simulink model "LQR_1"  (R2022a)
settings: Solver=VariableStepAuto  StartTime=0.0  StopTime=60  RelTol=1e-3
values from neighbouring files (symbols this model uses):
  A = double(A)    [LQR.m]
  B = double(B)    [LQR.m]
undefined symbols (not defined in the file or in its folder): K
libraries: cstblocks x2, simulink x1
settings Model: Creator=Shiva  LastModifiedBy=Shiva

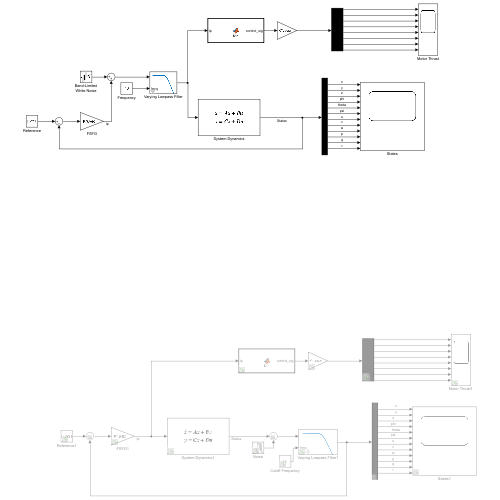
[thumbnail: Simulink's stored preview of the top-level diagram]
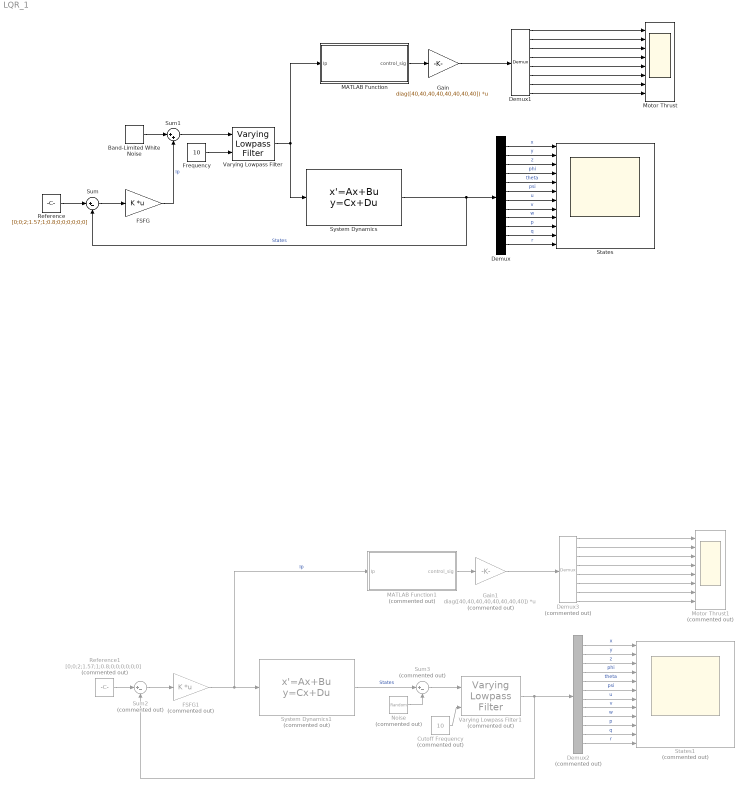
== system LQR_1 ==
  Band-Limited White Noise : simulink/Sources/Band-Limited White Noise  Cov=[0.1]  Ts=0.1  seed=[23341]
  Cutoff Frequency : Constant  Commented=on  Value=10
  Demux : Demux  Outputs=12
  Demux1 : Demux  Outputs=8
  Demux2 : Demux  Commented=on  Outputs=12
  Demux3 : Demux  Commented=on  Outputs=8
  FSFG : Gain  Gain=K  Multiplication=Matrix(K*u) (u vector)
  FSFG1 : Gain  Commented=on  Gain=K  Multiplication=Matrix(K*u) (u vector)
  Frequency : Constant  Value=10
  Gain : Gain  Gain=diag([40,40,40,40,40,40,40,40])  Multiplication=Matrix(K*u) (u vector)
  Gain1 : Gain  Commented=on  Gain=diag([40,40,40,40,40,40,40,40])  Multiplication=Matrix(K*u) (u vector)
  MATLAB Function : MATLAB Function  TreatAsAtomicUnit=on
  MATLAB Function1 : MATLAB Function  Commented=on  TreatAsAtomicUnit=on
  Motor Thrust : Scope  NumInputPorts=8
  Motor Thrust1 : Scope  Commented=on  NumInputPorts=8
  Noise : RandomNumber  Commented=on  Mean=[0 0 0 0 0 0 0.1 0.1 0.1 0 0 0]  Variance=[0 0 0 0 0 0 0.01 0.01 0.01 0 0 0]  SampleTime=0.1
  Reference : Constant  Value=[0;0;2;1.57;1;0.8;0;0;0;0;0;0]  SampleTime=-1
  Reference1 : Constant  Commented=on  Value=[0;0;2;1.57;1;0.8;0;0;0;0;0;0]  SampleTime=-1
  States : Scope  NumInputPorts=12
  States1 : Scope  Commented=on  NumInputPorts=12
  Sum : Sum  Inputs=|+-
  Sum1 : Sum  Inputs=|++
  Sum2 : Sum  Commented=on  Inputs=|+-
  Sum3 : Sum  Commented=on  Inputs=|+-
  System Dynamics : StateSpace  A=A  B=B  C=eye(12)  D=zeros(12,6)  InitialCondition=zeros(12,1)  ParameterTunability=Optimized
  System Dynamics1 : StateSpace  Commented=on  A=A  B=B  C=eye(12)  D=zeros(12,6)  InitialCondition=zeros(12,1)  ParameterTunability=Optimized
  Varying Lowpass Filter : cstblocks/Linear Parameter Varying/Varying Lowpass Filter  N=1
  Varying Lowpass Filter1 : cstblocks/Linear Parameter Varying/Varying Lowpass Filter  Commented=on  N=1
  wires:
  Reference/1 -> Sum/1
  System Dynamics/1 -> Sum/2, Demux/1  "States"
  Sum/1 -> FSFG/1
  Demux/1 -> States/1  "x"
  Demux/2 -> States/2  "y"
  Demux/3 -> States/3  "z"
  Demux/4 -> States/4  "phi"
  Demux/5 -> States/5  "theta"
  Demux/6 -> States/6  "psi"
  Demux/7 -> States/7  "u"
  Demux/8 -> States/8  "v"
  Demux/9 -> States/9  "w"
  Demux/10 -> States/10  "p"
  Demux/11 -> States/11  "q"
  Demux/12 -> States/12  "r"
  Demux1/1 -> Motor Thrust/1
  Demux1/2 -> Motor Thrust/2
  Demux1/3 -> Motor Thrust/3
  Demux1/4 -> Motor Thrust/4
  Demux1/5 -> Motor Thrust/5
  Demux1/6 -> Motor Thrust/6
  Demux1/7 -> Motor Thrust/7
  Demux1/8 -> Motor Thrust/8
  MATLAB Function/1(control_sig) -> Gain/1
  Gain/1 -> Demux1/1
  FSFG/1 -> Sum1/2  "Ip"
  Frequency/1 -> Varying Lowpass Filter/2
  Band-Limited White Noise/1 -> Sum1/1
  Sum1/1 -> Varying Lowpass Filter/1
  Varying Lowpass Filter/1 -> MATLAB Function/1(Ip), System Dynamics/1
  Demux3/8 -> Motor Thrust1/8
  Demux3/4 -> Motor Thrust1/4
  Gain1/1 -> Demux3/1
  Demux2/10 -> States1/10  "p"
  Demux3/3 -> Motor Thrust1/3
  Demux2/12 -> States1/12  "r"
  Demux2/7 -> States1/7  "u"
  Demux3/1 -> Motor Thrust1/1
  Reference1/1 -> Sum2/1
  Demux3/2 -> Motor Thrust1/2
  Sum2/1 -> FSFG1/1
  Demux3/5 -> Motor Thrust1/5
  MATLAB Function1/1(control_sig) -> Gain1/1
  Demux3/6 -> Motor Thrust1/6
  Demux2/6 -> States1/6  "psi"
  Demux2/5 -> States1/5  "theta"
  Demux3/7 -> Motor Thrust1/7
  Demux2/3 -> States1/3  "z"
  Demux2/8 -> States1/8  "v"
  Demux2/11 -> States1/11  "q"
  Demux2/2 -> States1/2  "y"
  Demux2/9 -> States1/9  "w"
  Demux2/4 -> States1/4  "phi"
  Demux2/1 -> States1/1  "x"
  FSFG1/1 -> System Dynamics1/1, MATLAB Function1/1(Ip)  "Ip"
  System Dynamics1/1 -> Sum3/1  "States"
  Noise/1 -> Sum3/2
  Sum3/1 -> Varying Lowpass Filter1/1
  Cutoff Frequency/1 -> Varying Lowpass Filter1/2
  Varying Lowpass Filter1/1 -> Sum2/2, Demux2/1

== matlab function LQR_1/MATLAB Function ==
  data: Ip input; control_sig output
function control_sig = fcn(Ip)
T=[0.707,0.707,-0.707,-0.707,0,0,0,0;
   -0.707,0.707,-0.707,0.707,0,0,0,0;
   0,0,0,0,-1,1,1,-1;
   0.06,-0.06,0.06,-0.06,-0.218,-0.218,0.218,0.218;
   0.06,0.06,-0.06,-0.06,0.120,-0.120,0.120,-0.120;
   -0.1888,0.1888,0.1888,-0.1888,0,0,0,0];

K=diag([40,40,40,40,40,40,40,40]);

T_star=(T.')*inv(T*(T.'));

control_sig=inv(K)*T_star*Ip;

== matlab function LQR_1/MATLAB Function1 ==
  data: Ip input; control_sig output
function control_sig = fcn(Ip)
T=[0.707,0.707,-0.707,-0.707,0,0,0,0;
   -0.707,0.707,-0.707,0.707,0,0,0,0;
   0,0,0,0,-1,1,1,-1;
   0.06,-0.06,0.06,-0.06,-0.218,-0.218,0.218,0.218;
   0.06,0.06,-0.06,-0.06,0.120,-0.120,0.120,-0.120;
   -0.1888,0.1888,0.1888,-0.1888,0,0,0,0];

K=diag([40,40,40,40,40,40,40,40]);

T_star=(T.')*inv(T*(T.'));

control_sig=inv(K)*T_star*Ip;
